simulink model "test_mppt_ic"  (R2020a)
settings: Solver=VariableStepAuto  StartTime=0.0  StopTime=2.5  RelTol=1e-3
libraries: powerlib x16, re_lib x4, powerlib_meascontrol x1
settings Model: Creator=Sanjayitha Raja  LastModifiedBy=Sanjayitha Raja

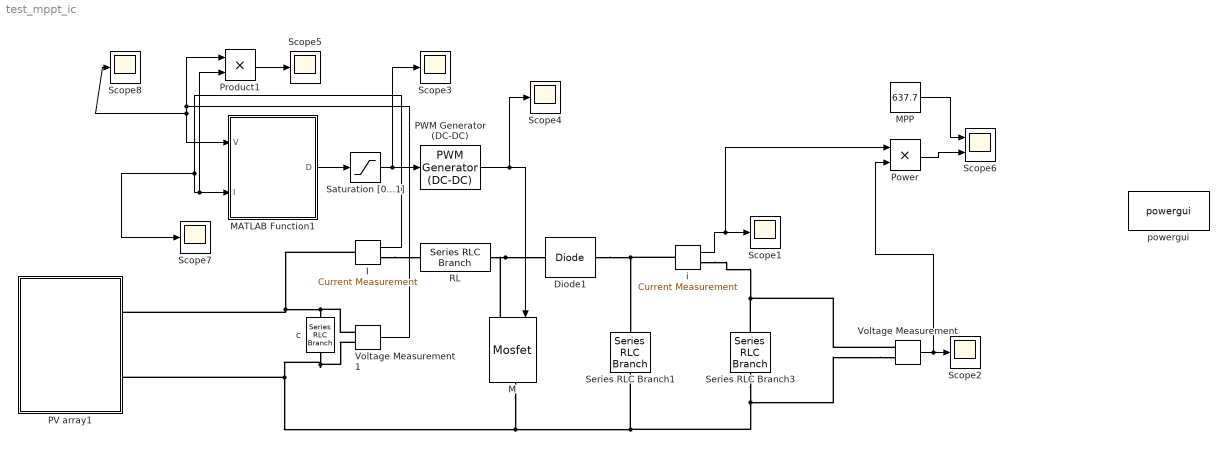
== system test_mppt_ic ==
  Diode1 : powerlib/Power Electronics/Diode  Ron=1e-3  Lon=0  Vf=0  IC=0  UseSnubber=off  Rs=inf  Cs=inf  Measurements=off
  I : powerlib/Measurements/Current Measurement  PhasorSimulation=off  OutputType=Magnitude  PSBequivalent=0
  M : powerlib/Power Electronics/Mosfet  Ron=1e-3  Lon=0  Rd=1e-3  Vfd=0  IC=0  Rs=inf  Cs=inf  Measurements=off
  MATLAB Function1 : MATLAB Function  TreatAsAtomicUnit=on
  MPP : Constant  Value=637.7
  PV array1 : Subsystem
  PWM Generator (DC-DC) : powerlib_meascontrol/Pulse & Signal Generators/PWM Generator (DC-DC)  Fsw=50e3  Ts=0
  Power : Product
  Product1 : Product
  RL : powerlib/Elements/Series RLC Branch  LConnTagsString=__new0  RConnTagsString=__new0  BranchType=L  Resistance=1e-3  Inductance=1.1478e-3  SetiL0=off  InitialCurrent=0  Capacitance=1e-6  Setx0=off  InitialVoltage=0  Measurements=None
  Saturation [0...1] : Saturate  UpperLimit=1  LowerLimit=0
  Scope{1..5,7..8} (7 alike) : Scope
  Scope6 : Scope  NumInputPorts=2
  Series RLC Branch1 : powerlib/Elements/Series RLC Branch  LConnTagsString=__new0  RConnTagsString=__new0  BranchType=C  Resistance=1e-4  Inductance=200e-6  SetiL0=off  InitialCurrent=0  Capacitance=0.4676e-3  Setx0=off  InitialVoltage=40  Measurements=None
  Series RLC Branch3 : powerlib/Elements/Series RLC Branch  LConnTagsString=__new0  RConnTagsString=__new0  BranchType=R  Resistance=53  Inductance=200e-6  SetiL0=off  InitialCurrent=0  Capacitance=1000e-6  Setx0=off  InitialVoltage=40  Measurements=None
  Voltage Measurement : powerlib/Measurements/Voltage Measurement  PhasorSimulation=off  OutputType=Magnitude  PSBequivalent=0
  Voltage Measurement1 : powerlib/Measurements/Voltage Measurement  PhasorSimulation=off  OutputType=Magnitude  PSBequivalent=0
  c : powerlib/Elements/Series RLC Branch  LConnTagsString=__new0  RConnTagsString=__new0  BranchType=C  Resistance=1e-3  Inductance=250e-6  SetiL0=off  InitialCurrent=0  Capacitance=10e-6  Setx0=off  InitialVoltage=0  Measurements=None
  i : powerlib/Measurements/Current Measurement  PhasorSimulation=off  OutputType=Magnitude  PSBequivalent=0
  powergui : powerlib/powergui  Priority=1  SimulationMode=Continuous  SampleTime=50e-6  frequency=60  Iterations=50  frequencyindice=0  Pbase=100e6  ErrMax=1e-4  UnitsV=kV  UnitsW=MW  buscounter=0  FunctionMessages=off  echomessages=off  EnableUseOfTLC=off  CurrentSourceSwitches=off  DisableSnubberDevices=off  DisableRonSwitches=off  DisableVfSwitches=off  DisplayEquations=off  AutomaticDiscreteSolvers=off  SolverType=Tustin/Backward Euler (TBE)  Interpol=off  ExternalGateDelay=off  methode=off  Ts=100  x0status=blocks  SPID=on  SwTol=0  HookPort=off  NonlinearTolerance=1e-4  nMaxIteration=100  ContinueOnMaxIteration=off  RestoreLinks=warning  ResistiveCurrentMeasurement=off  Frange=[0:2:500]  Ylog=off  Xlog=on  ShowGrid=off  save=off  variable=ZData  structure=0  ZoomFFT=off  StartTime=0.0  cycles=1  DisplayStyle=1  fundamental=60  FreqAxis=off  MaxFrequency=1000  frequencyindicesteady=1  RmsSteady=1  display=off
  wires:
  MPP/1 -> Scope6/1
  Power/1 -> Scope6/2
  Product1/1 -> Scope5/1
  i/1 -> Power/1, Scope1/1
  Voltage Measurement1/1 -> MATLAB Function1/1(V), Scope8/1, Product1/1
  Saturation [0...1]/1 -> Scope3/1, PWM Generator (DC-DC)/1
  MATLAB Function1/1(D) -> Saturation [0...1]/1
  I/1 -> MATLAB Function1/2(I), Product1/2, Scope7/1
  PWM Generator (DC-DC)/1 -> Scope4/1, M/1
  Voltage Measurement/1 -> Power/2, Scope2/1
  connections:
  i/LConn1 -- Diode1/RConn1 -- Series RLC Branch1/LConn1
  RL/RConn1 -- Diode1/LConn1 -- M/LConn1
  Voltage Measurement/LConn2 -- Series RLC Branch1/RConn1 -- Voltage Measurement1/LConn2 -- c/RConn1 -- PV array1/RConn2 -- M/RConn1 -- Series RLC Branch3/RConn1
  I/LConn1 -- c/LConn1 -- Voltage Measurement1/LConn1 -- PV array1/RConn1
  Voltage Measurement/LConn1 -- i/RConn1 -- Series RLC Branch3/LConn1
  I/RConn1 -- RL/LConn1

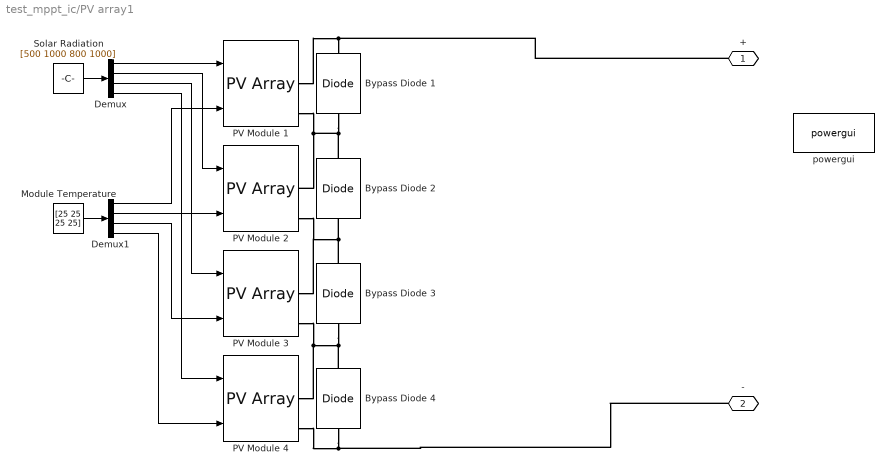
== system test_mppt_ic/PV array1 ==
  Bypass Diode {1..4} (4 alike) : powerlib/Power Electronics/Diode  Ron=0.001  Lon=0  Vf=0.8  IC=0  UseSnubber=off  Rs=500  Cs=250e-9  Measurements=off
  Demux : Demux
  Demux1 : Demux
  Module Temperature : Constant  Value=[25 25 25 25]
  PV Module {1..4} (4 alike) : re_lib/Solar/PV Array  Npar=1  Nser=1  PlotType=array @ 1000 W/m2 & specified temperatures  S_vec="[ 1000  500  100 ]"  Temp_C_vec="[ 45 25  ]"  ModuleName=Tata Power Solar Systems TP250MBZ  PlotWhenSelected=off  Pm=249  Ncell=60  Voc=36.8  Isc=8.83  Vm=30  Im=8.3  beta_Voc_pc=-0.33  alpha_Isc_pc=0.063805  beta_Voc=-0.12144  alpha_Isc=0.005634  IL=8.8382  I0=1.0132e-10  nI=0.94812  Rsh=314.7646  Rs=0.2914  RobustModel=off  RobustCellTemperature=25  BAL=off  Tc=1e-6  Tfilter=5e-5
  Solar Radiation : Constant  Value=[500 1000 800 1000]
  powergui : powerlib/powergui  Priority=1  SimulationMode=Continuous  SampleTime=50e-6  frequency=60  Iterations=50  frequencyindice=0  Pbase=100e6  ErrMax=1e-4  UnitsV=kV  UnitsW=MW  buscounter=0  FunctionMessages=off  echomessages=off  EnableUseOfTLC=off  CurrentSourceSwitches=off  DisableSnubberDevices=off  DisableRonSwitches=off  DisableVfSwitches=off  DisplayEquations=off  AutomaticDiscreteSolvers=off  SolverType=Tustin/Backward Euler (TBE)  Interpol=off  ExternalGateDelay=off  methode=off  Ts=100  x0status=blocks  SPID=on  SwTol=0  HookPort=off  NonlinearTolerance=1e-4  nMaxIteration=100  ContinueOnMaxIteration=off  RestoreLinks=warning  ResistiveCurrentMeasurement=off  Frange=[0:2:500]  Ylog=off  Xlog=on  ShowGrid=off  save=off  variable=ZData  structure=0  ZoomFFT=off  StartTime=0.0  cycles=1  DisplayStyle=1  fundamental=60  FreqAxis=off  MaxFrequency=1000  frequencyindicesteady=1  RmsSteady=1  display=off
  + : PMIOPort  Side=Right
  - : PMIOPort  Port=2  Side=Right
  wires:
  Solar Radiation/1 -> Demux/1
  Demux1/4 -> PV Module 4/2
  Demux/2 -> PV Module 2/1
  Module Temperature/1 -> Demux1/1
  Demux/3 -> PV Module 3/1
  Demux1/2 -> PV Module 2/2
  Demux/1 -> PV Module 1/1
  Demux1/1 -> PV Module 1/2
  Demux1/3 -> PV Module 3/2
  Demux/4 -> PV Module 4/1
  connections:
  Bypass Diode 3/RConn1 -- Bypass Diode 2/LConn1 -- PV Module 2/RConn2 -- PV Module 3/RConn1
  PV Module 3/RConn2 -- Bypass Diode 4/RConn1 -- Bypass Diode 3/LConn1 -- PV Module 4/RConn1
  Bypass Diode 2/RConn1 -- Bypass Diode 1/LConn1 -- PV Module 2/RConn1 -- PV Module 1/RConn2
  PV Module 1/RConn1 -- +/RConn1 -- Bypass Diode 1/RConn1
  Bypass Diode 4/LConn1 -- -/RConn1 -- PV Module 4/RConn2

== matlab function test_mppt_ic/MATLAB Function1 ==
  settings: updateMethod=DISCRETE  sampleTime=1e-4
  data: V input; D output; I input
% author : Mohamed LOUZAZNI
% National School of Applied Sciences, Tanger, Morocco
% f=10000 Hz (G)
function D=ModINC(V, I)


Dinit = 0.4;  %Initial value for D output
Dmax = 0.65;   %Maximum value for D
Dmin = 0.1;   %Minimum value for D
deltaD = 0.001; %Increment value used to increase/decrease the duty cycle D

  
persistent Vold Pold Dold M Iold;

dataType = 'double';

if isempty(Vold)
    Vold=0;
    Pold=0;
    Iold=0;
    Dold=Dinit;
 %   M=1;
end
P= V*I;
dV= V - Vold;
dP= P - Pold;
dI= I - Iold;
M=abs(dP);

if M < 0.005
    D=Dold;
else
    if dV == 0
        if dI == 0
            D=Dold;
        elseif dI>0
            D=Dold - (M*deltaD);
        else 
            D=Dold + (M*deltaD);
        end    
    else
        if dI/dV == -I/V
            D=Dold;
        elseif dI/dV>-I/V    
           D=Dold - (M*deltaD);
        else
           D=Dold + (M*deltaD);  
        end  
    end    
end

if D >= Dmax || D<= Dmin
    D=Dold;
end

Dold=D;
Vold=V;
Pold=P;
Iold=I;
